simulink model "linearized_anti_disturbance"  (R2016b)
settings: Solver=VariableStepAuto  StartTime=0.0  StopTime=10.0  RelTol=1e-3
values from neighbouring files (symbols this model uses):
  A = simplify(A)    [symbolic_rotor.m]
  C = [0,0,0,-L*mg*cos(beta)*beta_dot;0,0,0,L*mg*sin(beta)*beta_dot;0,0,0,0;0,0,0,0]    [disturbance_compensation_nonlinear_test.m]    (also in symbolic_rotor.m = [1,0,0,0, 0,0,0,0; uav_grasp_opt.m = [0,0,L*mg*sin(theta)*theta_dot;0,0,L*mg*cos(theta)*theta_dot; uav_grasp_opt_var_mass.m)
  K_z_arm = B_arm\E_arm    [disturbance_compensation.m]    (also in disturbance_compensation_nonlinear_test.m)
  K_z_drone = B_drone\E_drone    [disturbance_compensation.m]    (also in disturbance_compensation_nonlinear_test.m)
  V_arm = inv(C_arm*((B_arm*K_arm-A_arm)\B_arm))    [disturbance_compensation.m]    (also in disturbance_compensation_nonlinear_test.m)
  V_drone = inv(C_drone*((B_drone*K_drone-A_drone)\B_drone))    [disturbance_compensation.m]    (also in disturbance_compensation_nonlinear_test.m)
  x0 = zeros(8,1)    [decoupling_falb_wolovich.m]    (also in disturbance_compensation.m; disturbance_compensation_nonlinear_test.m = [0;0;0;pi/2;0;0;0;0]; riccati_controller_linear.m; symbolic_rotor.m)
undefined symbols (not defined in the file or in its folder): B_dbth, K_arm, K_drone
settings Model: Creator=Administrator  LastModifiedBy=Administrator

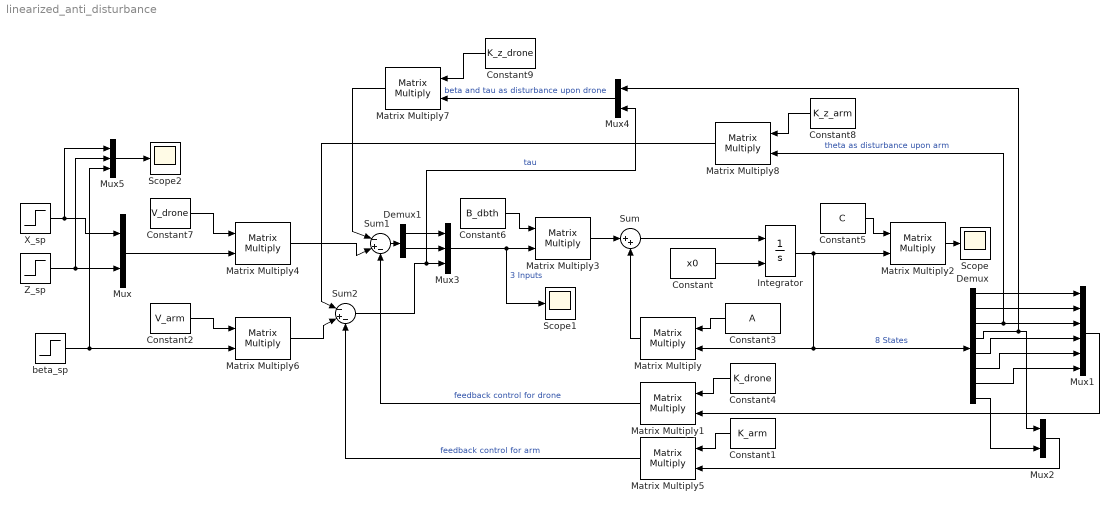
== system linearized_anti_disturbance ==
  Constant : Constant  Value=x0
  Constant1 : Constant  Value=K_arm  VectorParams1D=off
  Constant2 : Constant  Value=V_arm
  Constant3 : Constant  Value=A
  Constant4 : Constant  Value=K_drone
  Constant5 : Constant  Value=C
  Constant6 : Constant  Value=B_dbth
  Constant7 : Constant  Value=V_drone
  Constant8 : Constant  Value=K_z_arm
  Constant9 : Constant  Value=K_z_drone
  Demux : Demux  Outputs=8
  Demux1 : Demux  Outputs=2
  Integrator : Integrator  InitialConditionSource=external
  Matrix Multiply{,1..8} (9 alike) : Product  Multiplication=Matrix(*)
  Mux : Mux  Inputs=2
  Mux1 : Mux  Inputs=6
  Mux2 : Mux  Inputs=2
  Mux3 : Mux  Inputs=3
  Mux4 : Mux  Inputs=2
  Mux5 : Mux  Inputs=3
  Scope : Scope
  Scope1 : Scope
  Scope2 : Scope
  Sum : Sum  Inputs=|++
  Sum1 : Sum  Inputs=|-+-
  Sum2 : Sum  Inputs=|-+-
  X_sp : Step  SampleTime=0  VectorParams1D=off
  Z_sp : Step  SampleTime=0  VectorParams1D=off
  beta_sp : Step  Time=6  After=0.3  SampleTime=0  VectorParams1D=off
  wires:
  Constant/1 -> Integrator/2
  Sum/1 -> Integrator/1
  Integrator/1 -> Demux/1, Matrix Multiply/2, Matrix Multiply2/2  "8 States"
  Matrix Multiply/1 -> Sum/2
  Matrix Multiply3/1 -> Sum/1
  Matrix Multiply2/1 -> Scope/1
  Constant3/1 -> Matrix Multiply/1
  Mux/1 -> Matrix Multiply4/2
  Constant7/1 -> Matrix Multiply4/1
  Constant6/1 -> Matrix Multiply3/1
  Constant4/1 -> Matrix Multiply1/1
  Constant5/1 -> Matrix Multiply2/1
  X_sp/1 -> Mux5/1, Mux/1
  Z_sp/1 -> Mux5/2, Mux/2
  Demux/1 -> Mux1/1
  Demux/2 -> Mux1/2
  Demux/3 -> Mux1/3, Matrix Multiply8/2  "theta as disturbance upon arm"
  Demux/7 -> Mux1/6
  Demux/6 -> Mux1/5
  Demux/5 -> Mux1/4
  Demux/4 -> Mux4/1, Mux2/1
  Demux/8 -> Mux2/2
  Mux1/1 -> Matrix Multiply1/2
  Constant1/1 -> Matrix Multiply5/1
  Mux2/1 -> Matrix Multiply5/2
  Mux3/1 -> Scope1/1, Matrix Multiply3/2  "3 Inputs"
  Demux1/2 -> Mux3/2
  Demux1/1 -> Mux3/1
  Matrix Multiply4/1 -> Sum1/2
  Sum1/1 -> Demux1/1
  Matrix Multiply1/1 -> Sum1/3  "feedback control for drone"
  Sum2/1 -> Mux4/2, Mux3/3  "tau"
  Matrix Multiply5/1 -> Sum2/3  "feedback control for arm"
  beta_sp/1 -> Matrix Multiply6/2, Mux5/3
  Constant2/1 -> Matrix Multiply6/1
  Matrix Multiply6/1 -> Sum2/2
  Constant9/1 -> Matrix Multiply7/1
  Constant8/1 -> Matrix Multiply8/1
  Matrix Multiply8/1 -> Sum2/1
  Mux4/1 -> Matrix Multiply7/2  "beta and tau as disturbance upon drone"
  Matrix Multiply7/1 -> Sum1/1
  Mux5/1 -> Scope2/1
